simulink model "closedloop"  (R2018a)
settings: Solver=VariableStepAuto  StartTime=0.0  StopTime=10.0  RelTol=1e-3
undefined symbols (not defined in the file or in its folder): K
settings Model: Creator=kyniu  LastModifiedBy=kyniu

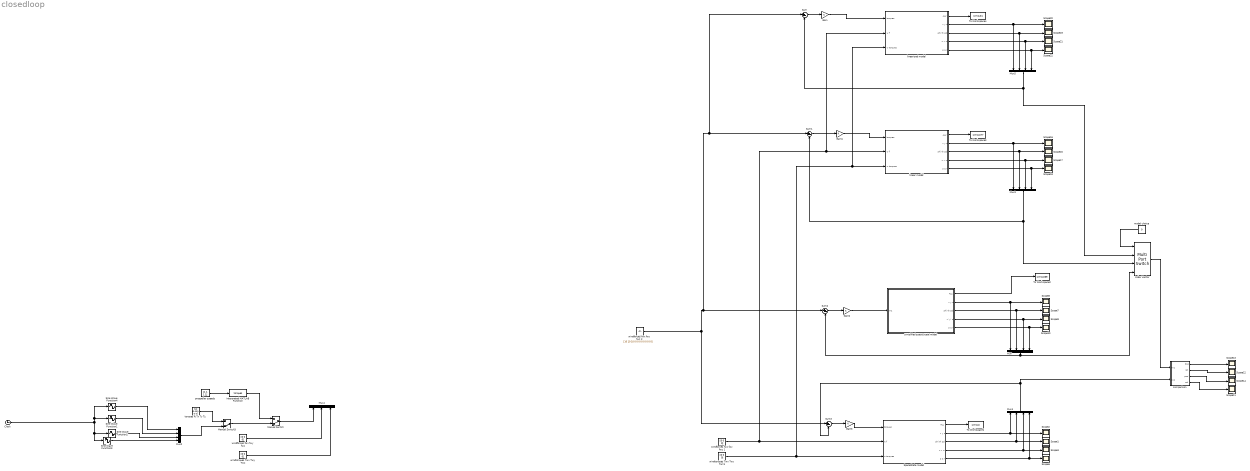
== system closedloop ==
  Clock : Clock
  Gain{,1..3} (4 alike) : Gain  Gain=K
  Index Vector : MultiPortSwitch  DataPortOrder=Zero-based contiguous  zeroidx=on
  Interpreted MATLAB Function : MATLABFcn  MATLABFcn=torques
  Manual Switch : ManualSwitch  CurrentSetting=0
  Manual Switch3 : ManualSwitch  CurrentSetting=0
  Mux{,1,3,5} (4 alike) : Mux  Inputs=[3 3 3 3]
  Mux2 : Mux
  Mux4 : Mux  Inputs=3
  Scope{1..3,6..22} (20 alike) : Scope
  Sine Wave Function1 : Sin  TimeSource=Use external signal  Amplitude=0.05  Frequency=6  SampleTime=0
  Sine Wave Function2 : Sin  TimeSource=Use external signal  Amplitude=0  SampleTime=0
  Sine Wave Function3 : Sin  TimeSource=Use external signal  Amplitude=0  Frequency=0.3  SampleTime=0
  Sine Wave Function4 : Sin  TimeSource=Use external signal  Amplitude=0  Bias=10  Frequency=6  SampleTime=0
  SpaceState model : Subsystem
  Sum{,1..3} (4 alike) : Sum  Inputs=|+-
  To Workspace1 : ToWorkspace  VariableName=simout  SaveFormat=Timeseries  SampleTime=-1
  To Workspace2 : ToWorkspace  VariableName=simout69  SaveFormat=Timeseries  SampleTime=-1
  To Workspace3 : ToWorkspace  VariableName=simout77  SaveFormat=Timeseries  SampleTime=-1
  To Workspace4 : ToWorkspace  VariableName=simout1  SaveFormat=Timeseries  SampleTime=-1
  comparison : Subsystem
  linear model : Subsystem
  linearised model : Subsystem
  model choice : Constant  Value=0
  proppeller speeds : Constant  Value=[1 1 1 1]
  simplified space state model : Subsystem
  torques ft Tx Ty Tz : Constant  Value=[10 0.001 0 0]
  "windforces fwx fwy fwz " : Constant  Value=[0 0 0]
  windforces fwx fwy fwz 1 : Constant  Value=[0 0 0]
  windforces fwx fwy fwz 2 : Constant  Value=[10 10 10 0 0 0 0 0 0 0 0 0]
  windtorques Twx Twy Twz : Constant  Value=[0 0 0]
  windtorques Twx Twy Twz1 : Constant  Value=[0 0 0]
  wires:
  proppeller speeds/1 -> Interpreted MATLAB Function/1
  Manual Switch/1 -> Mux4/1
  SpaceState model/2(x y z) -> Scope2/1, Mux1/1
  windtorques Twx Twy Twz/1 -> Mux4/3
  SpaceState model/1(ALL') -> To Workspace1/1
  SpaceState model/4(u v w) -> Scope3/1, Mux1/3
  SpaceState model/5(p q r) -> Scope6/1, Mux1/4
  SpaceState model/3(phi th psi) -> Scope1/1, Mux1/2
  "windforces fwx fwy fwz "/1 -> Mux4/2
  Interpreted MATLAB Function/1 -> Manual Switch/1
  Index Vector/1 -> comparison/1(In1)
  Mux3/1 -> Sum1/2, Index Vector/3
  Sine Wave Function3/1 -> Mux2/4
  linearised model/4(u v w) -> Scope21/1, Mux5/3
  linearised model/2(x y z) -> Scope20/1, Mux5/1
  linearised model/5(p q r) -> Scope22/1, Mux5/4
  linearised model/1(ALL') -> To Workspace4/1
  linear model/3(phi th psi) -> Scope15/1, Mux3/2
  linear model/1(ALL') -> To Workspace3/1
  linear model/5(p q r) -> Scope18/1, Mux3/4
  linear model/2(x y z) -> Scope16/1, Mux3/1
  torques ft Tx Ty Tz/1 -> Manual Switch3/1
  Mux/1 -> Index Vector/4, Sum2/2
  comparison/4(rot') -> Scope11/1
  Mux1/1 -> Sum3/2, comparison/2(In2)
  comparison/2(rot) -> Scope12/1
  Mux2/1 -> Manual Switch3/2
  Manual Switch3/1 -> Manual Switch/2
  Mux5/1 -> Sum/2, Index Vector/2
  model choice/1 -> Index Vector/1
  Sine Wave Function2/1 -> Mux2/3
  comparison/1(Pos) -> Scope13/1
  linearised model/3(phi th psi) -> Scope19/1, Mux5/2
  simplified space state model/5(p q r) -> Mux/4, Scope10/1
  simplified space state model/3(phi th psi) -> Scope7/1, Mux/2
  simplified space state model/1(ALL') -> To Workspace2/1
  simplified space state model/2(x y z) -> Scope8/1, Mux/1
  linear model/4(u v w) -> Scope17/1, Mux3/3
  Sine Wave Function4/1 -> Mux2/1
  Clock/1 -> Sine Wave Function3/1, Sine Wave Function2/1, Sine Wave Function4/1, Sine Wave Function1/1
  simplified space state model/4(x' y' z') -> Scope9/1, Mux/3
  comparison/3(pos') -> Scope14/1
  Sine Wave Function1/1 -> Mux2/2
  windforces fwx fwy fwz 1/1 -> linearised model/2(w f), linear model/2(w f), SpaceState model/2(w f)
  windtorques Twx Twy Twz1/1 -> linearised model/3(w torques), linear model/3(w torques), SpaceState model/3(w torques)
  Sum/1 -> Gain/1
  Sum1/1 -> Gain1/1
  Sum2/1 -> Gain2/1
  Sum3/1 -> Gain3/1
  windforces fwx fwy fwz 2/1 -> Sum3/1, Sum/1, Sum1/1, Sum2/1
  Gain/1 -> linearised model/1(torques)
  Gain1/1 -> linear model/1(torques)
  Gain2/1 -> simplified space state model/1(In1)
  Gain3/1 -> SpaceState model/1(torques)

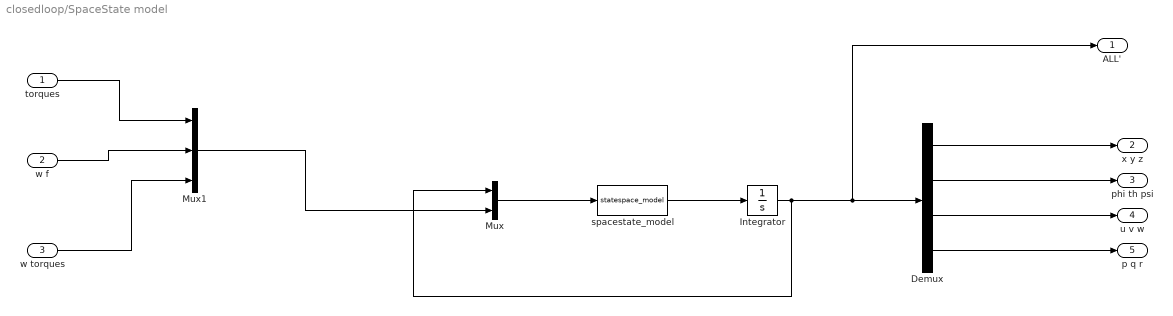
== system closedloop/SpaceState model ==
  torques : Inport
  w f : Inport  Port=2
  w torques : Inport  Port=3
  Demux : Demux  Outputs=[3 3 3 3]
  Integrator : Integrator  InitialCondition=[0 0 0 0 0 0 0 0 0 0 0 0]
  Mux : Mux  Inputs=2
  Mux1 : Mux  Inputs=3
  spacestate_model : MATLABFcn  MATLABFcn=statespace_model
  ALL' : Outport
  x y z : Outport  Port=2
  phi th psi : Outport  Port=3
  u v w : Outport  Port=4
  p q r : Outport  Port=5
  wires:
  Integrator/1 -> ALL'/1, Demux/1, Mux/1
  Demux/1 -> x y z/1
  Mux1/1 -> Mux/2
  torques/1 -> Mux1/1
  Mux/1 -> spacestate_model/1
  spacestate_model/1 -> Integrator/1
  Demux/4 -> p q r/1
  w f/1 -> Mux1/2
  w torques/1 -> Mux1/3
  Demux/2 -> phi th psi/1
  Demux/3 -> u v w/1

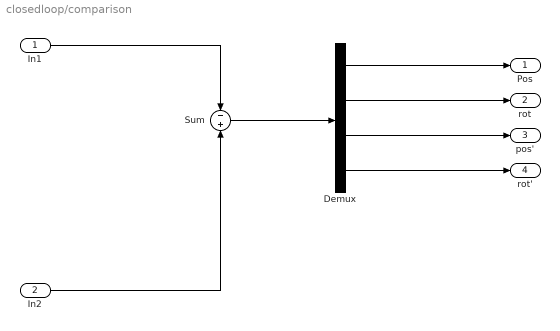
== system closedloop/comparison ==
  In1 : Inport
  In2 : Inport  Port=2
  Demux : Demux  Outputs=[3 3 3 3]
  Sum : Sum  Inputs=-+
  Pos : Outport
  rot : Outport  Port=2
  pos' : Outport  Port=3
  rot' : Outport  Port=4
  wires:
  Sum/1 -> Demux/1
  In1/1 -> Sum/1
  Demux/2 -> rot/1
  Demux/3 -> pos'/1
  In2/1 -> Sum/2
  Demux/1 -> Pos/1
  Demux/4 -> rot'/1

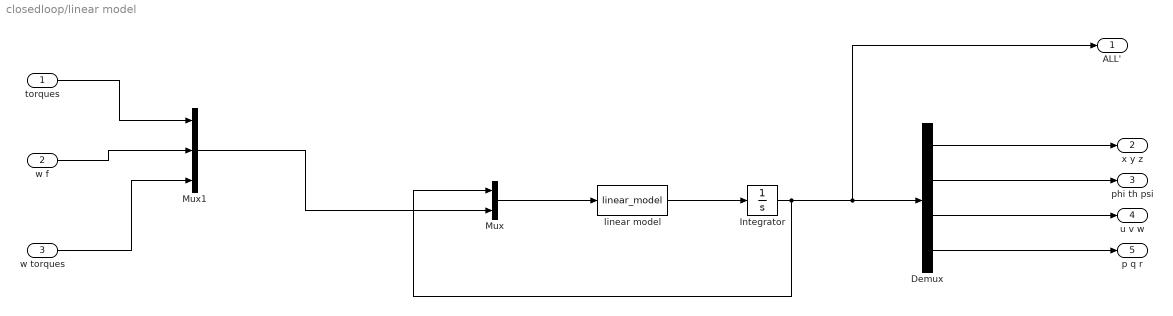
== system closedloop/linear model ==
  torques : Inport
  w f : Inport  Port=2
  w torques : Inport  Port=3
  Demux : Demux  Outputs=[3 3 3 3]
  Integrator : Integrator  InitialCondition=[0 0 0 0 0 0 0 0 0 0 0 0]
  Mux : Mux  Inputs=2
  Mux1 : Mux  Inputs=3
  linear model : MATLABFcn  MATLABFcn=linear_model
  ALL' : Outport
  x y z : Outport  Port=2
  phi th psi : Outport  Port=3
  u v w : Outport  Port=4
  p q r : Outport  Port=5
  wires:
  Integrator/1 -> ALL'/1, Demux/1, Mux/1
  Demux/1 -> x y z/1
  Mux1/1 -> Mux/2
  torques/1 -> Mux1/1
  Mux/1 -> linear model/1
  linear model/1 -> Integrator/1
  Demux/4 -> p q r/1
  w f/1 -> Mux1/2
  w torques/1 -> Mux1/3
  Demux/2 -> phi th psi/1
  Demux/3 -> u v w/1

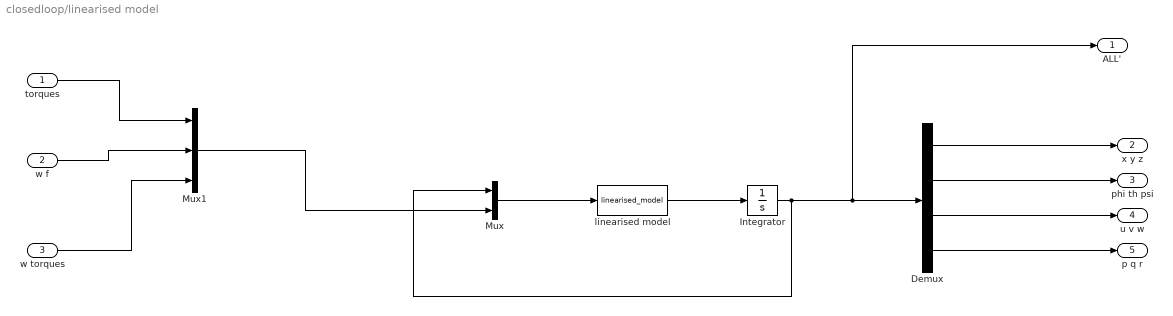
== system closedloop/linearised model ==
  torques : Inport
  w f : Inport  Port=2
  w torques : Inport  Port=3
  Demux : Demux  Outputs=[3 3 3 3]
  Integrator : Integrator  InitialCondition=[0 0 0 0 0 0 0 0 0 0 0 0]
  Mux : Mux  Inputs=2
  Mux1 : Mux  Inputs=3
  linearised model : MATLABFcn  MATLABFcn=linearised_model
  ALL' : Outport
  x y z : Outport  Port=2
  phi th psi : Outport  Port=3
  u v w : Outport  Port=4
  p q r : Outport  Port=5
  wires:
  Integrator/1 -> ALL'/1, Demux/1, Mux/1
  Demux/1 -> x y z/1
  Mux1/1 -> Mux/2
  torques/1 -> Mux1/1
  Mux/1 -> linearised model/1
  linearised model/1 -> Integrator/1
  Demux/4 -> p q r/1
  w f/1 -> Mux1/2
  w torques/1 -> Mux1/3
  Demux/2 -> phi th psi/1
  Demux/3 -> u v w/1

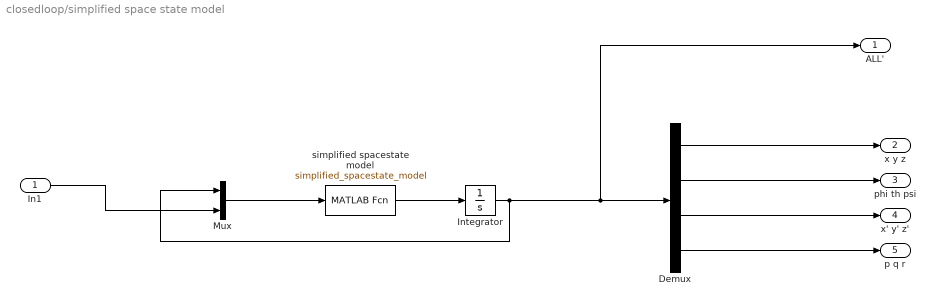
== system closedloop/simplified space state model ==
  In1 : Inport
  Demux : Demux  Outputs=[3 3 3 3]
  Integrator : Integrator  InitialCondition=[0 0 0 0 0 0 0 0 0 0 0 0]
  Mux : Mux  Inputs=2
  simplified spacestate model : MATLABFcn  MATLABFcn=simplified_spacestate_model
  ALL' : Outport
  x y z : Outport  Port=2
  phi th psi : Outport  Port=3
  x' y' z' : Outport  Port=4
  p q r : Outport  Port=5
  wires:
  Demux/3 -> x' y' z'/1
  Integrator/1 -> ALL'/1, Demux/1, Mux/1
  simplified spacestate model/1 -> Integrator/1
  In1/1 -> Mux/2
  Demux/4 -> p q r/1
  Demux/1 -> x y z/1
  Mux/1 -> simplified spacestate model/1
  Demux/2 -> phi th psi/1
